simulink model "DigitalTwin_withMA_Mask"  (R2025b)
settings: Solver=VariableStepAuto  StartTime=0.0  StopTime=0.03  RelTol=1e-3
InitFcn:
  | KF_param
values from neighbouring files (symbols this model uses):
  Ae2 = [A2, BF ... (first row only)    [KF_param.m]
  BI = [BI_0; BI_i{1}; BI_i{2}; BI_i{3}; BI_i{4}; BI_i{5}; BI_i{6}]    [KF_param.m]
  c = [0.09 0.034 0.03 0.08 0.03 0.08 0.05 0.05]    [KF_param.m]
  Ce2 = [C2, 0]    [KF_param.m]
  CF2 = [0 0 0 0 0 0 0 0 0 0 0 0 0 0 1]    [KF_param.m]
  f = [198 188 51 67 98 138 273 450]    [KF_param.m]    (also in computeFRF.m = (0:floor(N/2)-1)*(fs/N))
  k = [2.9E+6 2.6E+6 -2.0E+6 -400000 -9.0E+6 -800000 4.0E+6 -950000]    [KF_param.m]
  K2 = [ 1.09e6     3.64e5    -5.29e-15   -4.91e-15 -5.57e-15  -9.63e-16  -8.43e-16   -2.71e-17 -2.40e-17   2.60e-15   4.71e-16    5.35e-16 -8.28e-16  -3.11e-15   6.32e10 ]'    [KF_param.m]
undefined symbols (not defined in the file or in its folder): CurrentAmplitude, CurrentFreqHz
libraries: simulink x7
settings Model: Creator=Tharun Kumar  LastModifiedBy=Lenovo
settings SimscapeCC: SimscapeLogDecimation=1  SimscapeLogDataHistory=5000

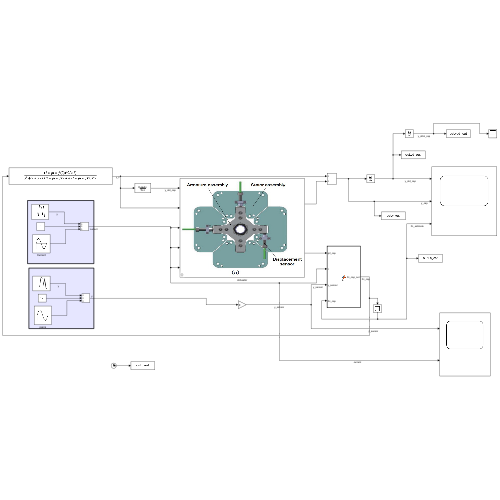
[thumbnail: Simulink's stored preview of the top-level diagram]
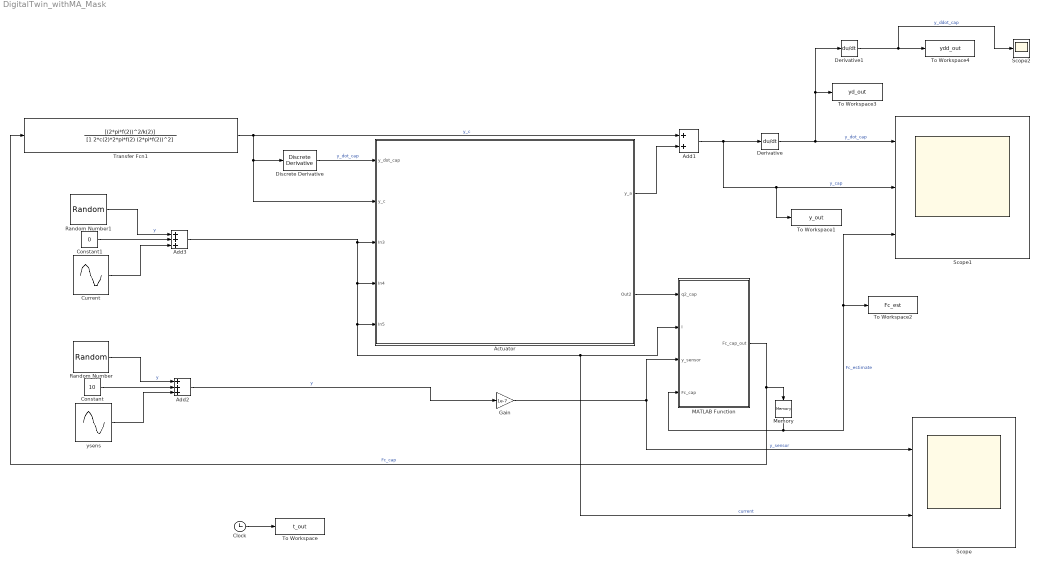
== system DigitalTwin_withMA_Mask ==
  Actuator : Subsystem
      mask Display:
      | text(5, 10, 'Actuator');
      | image('front.jpg');
  Add1 : Sum
  Add2 : Sum  Inputs=+++
  Add3 : Sum  Inputs=+++
  Clock : Clock
  Constant : Constant  Value=10
  Constant1 : Constant  Value=0
  Current : Sin  Amplitude=CurrentAmplitude  Frequency=CurrentFreqHz  SampleTime=0
  Derivative : Derivative
  Derivative1 : Derivative
  Discrete Derivative : simulink/Discrete/Discrete Derivative  gainval=1.0  ICPrevScaledInput=0.0  OutMin=[]  OutMax=[]  OutDataType=fixdt(1, 16)  OutScaling=2^-10  DoSatur=off
  Gain : Gain  Gain=1e-7
  MATLAB Function : MATLAB Function  TreatAsAtomicUnit=on
  Memory : Memory
  Random Number : RandomNumber  SampleTime=0.01
  Random Number1 : RandomNumber  SampleTime=0.01
  Scope : Scope  NumInputPorts=2
      settings: ActiveDisplayYMinimum=-1  ActiveDisplayYMaximum=1
  Scope1 : Scope  NumInputPorts=3
      settings: ActiveDisplayYMinimum=-1  ActiveDisplayYMaximum=1
  Scope2 : Scope
      settings: ActiveDisplayYMinimum=-1  ActiveDisplayYMaximum=1
  To Workspace : ToWorkspace  VariableName=t_out  SampleTime=-1
  To Workspace1 : ToWorkspace  VariableName=y_out  SampleTime=-1
  To Workspace2 : ToWorkspace  VariableName=Fc_est  SampleTime=-1
  To Workspace3 : ToWorkspace  VariableName=yd_out  SampleTime=-1
  To Workspace4 : ToWorkspace  VariableName=ydd_out  SampleTime=-1
  Transfer Fcn1 : TransferFcn  Numerator=[(2*pi*f(2))^2/k(2)]  Denominator=[1 2*c(2)*2*pi*f(2) (2*pi*f(2))^2]
  ysens : Sin  Amplitude=10  SampleTime=0
  wires:
  MATLAB Function/1(Fc_cap_out) -> Transfer Fcn1/1, Memory/1  "Fc_cap"
  Actuator/2(Out2) -> MATLAB Function/1(q2_cap)
  Actuator/1(y_a) -> Add1/2
  Memory/1 -> To Workspace2/1, Scope1/3, MATLAB Function/4(Fc_cap)  "Fc_estimate"
  Transfer Fcn1/1 -> Actuator/2(y_c), Discrete Derivative/1, Add1/1  "y_c"
  Discrete Derivative/1 -> Actuator/1(y_dot_cap)  "y_dot_cap"
  Add2/1 -> Gain/1  "y"
  Gain/1 -> Scope/1, MATLAB Function/3(y_sensor)  "y_sensor"
  Add1/1 -> Derivative/1, Scope1/2, To Workspace1/1  "y_cap"
  Derivative/1 -> Derivative1/1, To Workspace3/1, Scope1/1  "y_dot_cap"
  Random Number/1 -> Add2/1  "y"
  Constant/1 -> Add2/2
  ysens/1 -> Add2/3
  Random Number1/1 -> Add3/1  "y"
  Constant1/1 -> Add3/2
  Current/1 -> Add3/3
  Add3/1 -> Scope/2, MATLAB Function/2(I), Actuator/5(In5), Actuator/4(In4), Actuator/3(In3)  "current"
  Clock/1 -> To Workspace/1
  Derivative1/1 -> Scope2/1, To Workspace4/1  "y_ddot_cap"

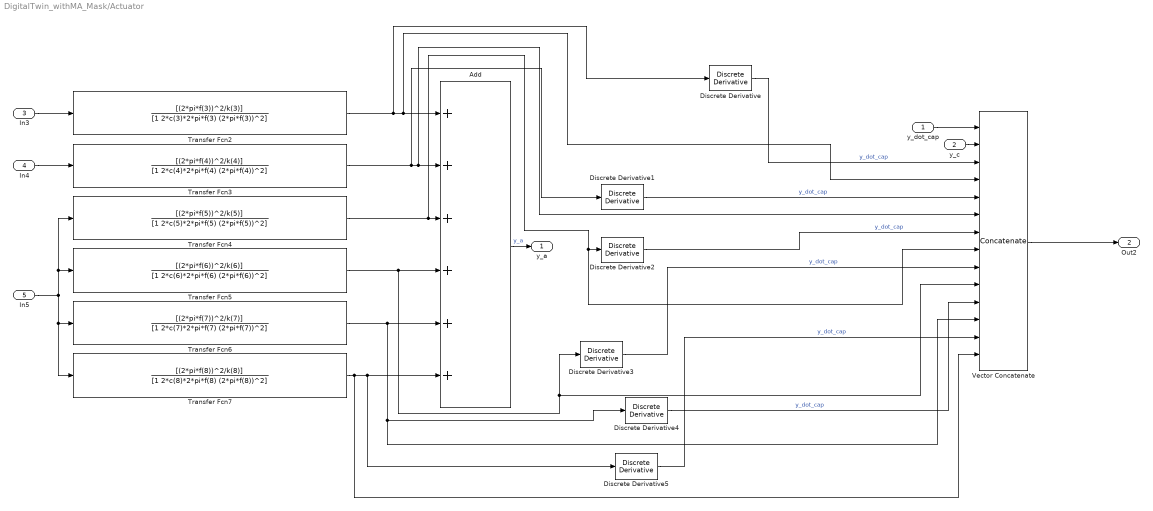
== system DigitalTwin_withMA_Mask/Actuator ==
  y_dot_cap : Inport
  y_c : Inport  Port=2
  In3 : Inport  Port=3
  In4 : Inport  Port=4
  In5 : Inport  Port=5
  Add : Sum  Inputs=++++++
  Discrete Derivative{,1..5} (6 alike) : simulink/Discrete/Discrete Derivative  gainval=1.0  ICPrevScaledInput=0.0  OutMin=[]  OutMax=[]  OutDataType=fixdt(1, 16)  OutScaling=2^-10  DoSatur=off
  Transfer Fcn2 : TransferFcn  Numerator=[(2*pi*f(3))^2/k(3)]  Denominator=[1 2*c(3)*2*pi*f(3) (2*pi*f(3))^2]
  Transfer Fcn3 : TransferFcn  Numerator=[(2*pi*f(4))^2/k(4)]  Denominator=[1 2*c(4)*2*pi*f(4) (2*pi*f(4))^2]
  Transfer Fcn4 : TransferFcn  Numerator=[(2*pi*f(5))^2/k(5)]  Denominator=[1 2*c(5)*2*pi*f(5) (2*pi*f(5))^2]
  Transfer Fcn5 : TransferFcn  Numerator=[(2*pi*f(6))^2/k(6)]  Denominator=[1 2*c(6)*2*pi*f(6) (2*pi*f(6))^2]
  Transfer Fcn6 : TransferFcn  Numerator=[(2*pi*f(7))^2/k(7)]  Denominator=[1 2*c(7)*2*pi*f(7) (2*pi*f(7))^2]
  Transfer Fcn7 : TransferFcn  Numerator=[(2*pi*f(8))^2/k(8)]  Denominator=[1 2*c(8)*2*pi*f(8) (2*pi*f(8))^2]
  Vector Concatenate : Concatenate  NumInputs=14
  y_a : Outport
  Out2 : Outport  Port=2
  wires:
  Transfer Fcn4/1 -> Vector Concatenate/8, Discrete Derivative2/1, Add/3
  Transfer Fcn3/1 -> Discrete Derivative1/1, Vector Concatenate/6, Add/2
  Discrete Derivative4/1 -> Vector Concatenate/11  "y_dot_cap"
  Transfer Fcn7/1 -> Discrete Derivative5/1, Add/6, Vector Concatenate/14
  In3/1 -> Transfer Fcn2/1
  In5/1 -> Transfer Fcn4/1, Transfer Fcn5/1, Transfer Fcn7/1, Transfer Fcn6/1
  y_c/1 -> Vector Concatenate/2
  In4/1 -> Transfer Fcn3/1
  Transfer Fcn2/1 -> Discrete Derivative/1, Add/1, Vector Concatenate/4
  Transfer Fcn5/1 -> Discrete Derivative3/1, Vector Concatenate/10, Add/4
  Discrete Derivative/1 -> Vector Concatenate/3  "y_dot_cap"
  Discrete Derivative5/1 -> Vector Concatenate/13  "y_dot_cap"
  Transfer Fcn6/1 -> Add/5, Discrete Derivative4/1, Vector Concatenate/12
  Add/1 -> y_a/1  "y_a"
  y_dot_cap/1 -> Vector Concatenate/1
  Vector Concatenate/1 -> Out2/1
  Discrete Derivative1/1 -> Vector Concatenate/5  "y_dot_cap"
  Discrete Derivative2/1 -> Vector Concatenate/7  "y_dot_cap"
  Discrete Derivative3/1 -> Vector Concatenate/9  "y_dot_cap"

== matlab function DigitalTwin_withMA_Mask/MATLAB Function ==
  data: q2_cap input; I input; y_sensor input; Fc_cap input; Ae2 parameter; K2 parameter; Ce2 parameter; CF2 parameter; BI parameter; Fc_cap_out output
function Fc_cap_out    = fcn(q2_cap, I, y_sensor, Fc_cap, Ae2,K2, Ce2, CF2, BI)


Bi=[BI;0];
qe2_cap = [q2_cap; Fc_cap];

qe2_cap = (Ae2-K2*Ce2)*qe2_cap +K2*y_sensor+Bi*I;

y_cap=sum(Ce2*qe2_cap,"all");

Fc_cap_out = CF2*qe2_cap;
